simulink model "brightnessController_Harness2"  (R2020b)
settings: Solver=VariableStepAuto  StartTime=0.0  StopTime=10.0  RelTol=1e-3
settings Model: Creator=Balazs  LastModifiedBy=Balazs

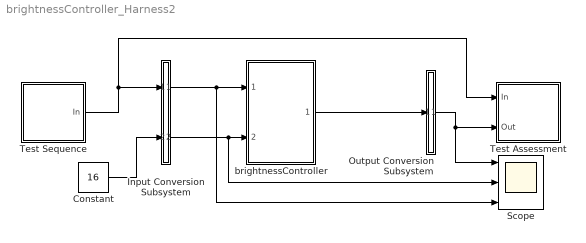
== system brightnessController_Harness2 ==
  Constant : Constant  Value=16  OutDataTypeStr=uint16
  Input Conversion Subsystem : Subsystem  Tag=__SLT_ICS__  Description=|
      | Signal spec.
      | and routing
      settings: AttributesFormatString=%<Description>
  Output Conversion Subsystem : Subsystem  Tag=__SLT_OCS__  Description=|
      | Signal spec.
      | and routing
      settings: AttributesFormatString=%<Description>
  Scope : Scope  NumInputPorts=3
  Test Assessment : Test Sequence  TreatAsAtomicUnit=on
  Test Sequence : Test Sequence  TreatAsAtomicUnit=on
  brightnessController : ModelReference  ModelNameDialog=brightnessController  SimulationMode=Normal  ModelReferenceVersion=1.11
  wires:
  Output Conversion Subsystem/1(Outport_1) -> Test Assessment/2(Out), Scope/1
  Input Conversion Subsystem/1(Outport_1) -> Scope/3, brightnessController/1
  Input Conversion Subsystem/2(Outport_2) -> Scope/2, brightnessController/2
  brightnessController/1 -> Output Conversion Subsystem/1(Inport_1)
  Test Sequence/1(In) -> Test Assessment/1(In), Input Conversion Subsystem/1(Inport_1)
  Constant/1 -> Input Conversion Subsystem/2(Inport_2)

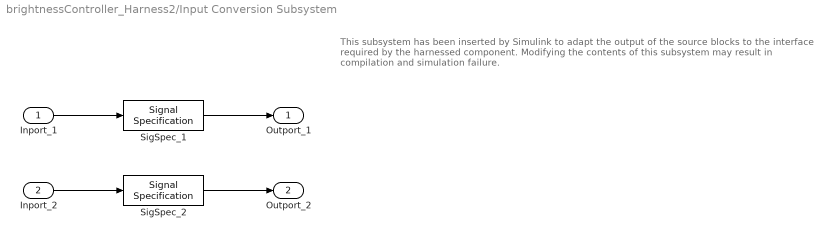
== system brightnessController_Harness2/Input Conversion Subsystem ==
  note: This subsystem has been inserted by Simulink to adapt the output of the source blocks to the interface required by the harnessed component.
      |  Modifying the contents of this subsystem may result in compilation and simulation failure.
  Inport_1 : Inport
  Inport_2 : Inport  Port=2
  SigSpec_1 : SignalSpecification  OutDataTypeStr=boolean  Dimensions=[1]  SampleTime=[0, 1]
  SigSpec_2 : SignalSpecification  OutDataTypeStr=uint16  Dimensions=[1]  SampleTime=[0, 1]
  Outport_1 : Outport
  Outport_2 : Outport  Port=2
  wires:
  SigSpec_1/1 -> Outport_1/1
  Inport_1/1 -> SigSpec_1/1
  SigSpec_2/1 -> Outport_2/1
  Inport_2/1 -> SigSpec_2/1

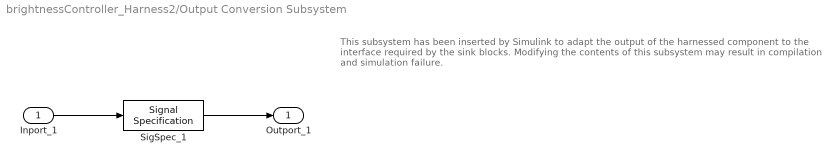
== system brightnessController_Harness2/Output Conversion Subsystem ==
  note: This subsystem has been inserted by Simulink to adapt the output of the harnessed component to the interface required by the sink blocks.
      |  Modifying the contents of this subsystem may result in compilation and simulation failure.
  Inport_1 : Inport
  SigSpec_1 : SignalSpecification  OutDataTypeStr=uint16  Dimensions=[1]
  Outport_1 : Outport
  wires:
  Inport_1/1 -> SigSpec_1/1
  SigSpec_1/1 -> Outport_1/1

== stateflow chart brightnessController_Harness2/Test Assessment ==
  settings: stateMachineType=SIMPLIFIED_MACHINE
  state Assessments
    Pulses = 0
    state CheckInit
      verify(Out == 0, 'Init error')
    state CheckPulse
      verify(Out == 4, 'Test failure')
    state Else
    Assessments -> (junction 22)
    (default) -> (junction 22)
    (junction 22) -> (junction 23) [order 1] : [et(sec)==0
        | ]
    (junction 23) -> CheckInit [order 1] : [~in(CheckInit)]
    (junction 22) -> (junction 31) [order 2]
    (junction 23) -> (junction 26) [order 2]
    (junction 31) -> (junction 32) [order 1] : [et(sec)==1
        | ]
    (junction 32) -> CheckPulse [order 1] : [~in(CheckPulse)]
    (junction 32) -> (junction 35) [order 2]
    (junction 45) -> (junction 46)
    (junction 46) -> Else [order 1] : [~in(Else)]
    (junction 46) -> (junction 49) [order 2]
    (junction 31) -> (junction 45) [order 2]
  (default) -> Assessments
  data: In input boolean; Out input uint16; Pulses local

== stateflow chart brightnessController_Harness2/Test Sequence ==
  settings: stateMachineType=SIMPLIFIED_MACHINE
  state Init
    In = false
  state PulseBegin
    In = true
  state PulseEnd
    In = false
  (default) -> Init
  Init -> PulseBegin : [
      | after(1,sec)
      | ]
  PulseBegin -> PulseEnd : [
      | after(1,sec)
      | ]
  data: In output boolean
